simulink model "teaching20260718"  (R2026a)
settings: Solver=VariableStepAuto
settings Model: Creator=itsyu  LastModifiedBy=itsyu

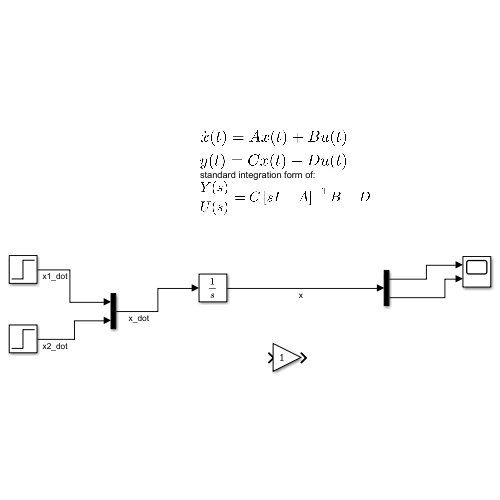
[thumbnail: Simulink's stored preview of the top-level diagram]
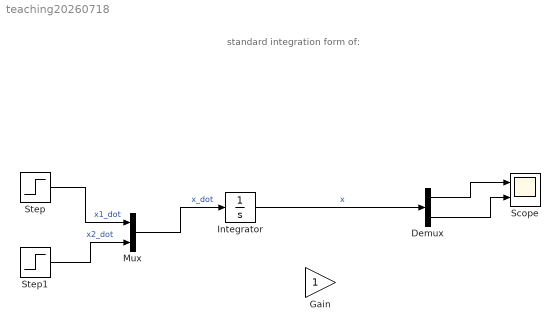
== system teaching20260718 ==
  note: standard integration form of:
  Demux : Demux  Outputs=2
  Gain : Gain
  Integrator : Integrator  InitialCondition=[0 0 ]
  Mux : Mux  Inputs=2
  Scope : Scope  NumInputPorts=2
      settings: ActiveDisplayYMinimum=-1.125  ActiveDisplayYMaximum=10.125000000000002
  Step : Step  SampleTime=0
  Step1 : Step  Time=3  SampleTime=0
  wires:
  Integrator/1 -> Demux/1  "x"
  Step/1 -> Mux/1  "x1_dot"
  Step1/1 -> Mux/2  "x2_dot"
  Mux/1 -> Integrator/1  "x_dot"
  Demux/1 -> Scope/1
  Demux/2 -> Scope/2
